simulink model "QD2_MissionCtrl_Swarm_6x_R2021a"  (R2021a)
settings: Solver=ode2  StartTime=0.0  StopTime=inf  FixedStep=0.001  RelTol=1e-3  EnableMultiTasking=on
undefined symbols (not defined in the file): datetime, Host, localhost, m, qc_get_step_size, saved_data
libraries: quarc_library x64, simulink x19, simulink_extras x1
(part 3 of 3)

== system QD2_MissionCtrl_Swarm_6x_R2021a/MISSION SERVER QDRONE SWARM/Calculate Home Pose V6/Enabled Subsystem ==
  "Pose (m, rad ) [4] " : Inport
  Enable : EnablePort
  "Home Pose (m, rad ) [4]" : Outport  VectorParamsAs1DForOutWhenUnconnected=off
  wires:
  "Pose (m, rad ) [4] "/1 -> "Home Pose (m, rad ) [4]"/1

== system QD2_MissionCtrl_Swarm_6x_R2021a/MISSION SERVER QDRONE SWARM/Calculate Home Pose V7/Enabled Subsystem ==
  "Pose (m, rad ) [4] " : Inport
  Enable : EnablePort
  "Home Pose (m, rad ) [4]" : Outport  VectorParamsAs1DForOutWhenUnconnected=off
  wires:
  "Pose (m, rad ) [4] "/1 -> "Home Pose (m, rad ) [4]"/1

== system QD2_MissionCtrl_Swarm_6x_R2021a/MISSION SERVER QDRONE SWARM/Communications Check/Triggered Subsystem ==
  note: This looks for the first falling edge to trigger a communication issue,
      | because the mission server model starts first.
  Trigger : TriggerPort  TriggerType=falling  VariantControl=Variant
  Add : Sum
  Compare To Constant : simulink/Logic and Bit Operations/Compare To Constant  relop=>=  const=1  OutDataTypeStr=boolean
  Constant : Constant
  Memory : Memory  InheritSampleTime=on
  Communication Issue (0,1) : Outport  InitialOutput=0  VectorParamsAs1DForOutWhenUnconnected=off
  wires:
  Constant/1 -> Add/1
  Memory/1 -> Add/2
  Add/1 -> Compare To Constant/1, Memory/1
  Compare To Constant/1 -> Communication Issue (0,1)/1

== system QD2_MissionCtrl_Swarm_6x_R2021a/MISSION SERVER QDRONE SWARM/Communications Check/Triggered Subsystem1 ==
  note: This looks for the first falling edge to trigger a communication issue,
      | because the mission server model starts first.
  Trigger : TriggerPort  TriggerType=falling  VariantControl=Variant
  Add : Sum
  Compare To Constant : simulink/Logic and Bit Operations/Compare To Constant  relop=>=  const=1  OutDataTypeStr=boolean
  Constant : Constant
  Memory : Memory  InheritSampleTime=on
  Communication Issue (0,1) : Outport  InitialOutput=0  VectorParamsAs1DForOutWhenUnconnected=off
  wires:
  Compare To Constant/1 -> Communication Issue (0,1)/1
  Add/1 -> Memory/1, Compare To Constant/1
  Memory/1 -> Add/2
  Constant/1 -> Add/1

== system QD2_MissionCtrl_Swarm_6x_R2021a/MISSION SERVER QDRONE SWARM/Communications Check/Triggered Subsystem2 ==
  note: This looks for the first falling edge to trigger a communication issue,
      | because the mission server model starts first.
  Trigger : TriggerPort  TriggerType=falling  VariantControl=Variant
  Add : Sum
  Compare To Constant : simulink/Logic and Bit Operations/Compare To Constant  relop=>=  const=1  OutDataTypeStr=boolean
  Constant : Constant
  Memory : Memory  InheritSampleTime=on
  Communication Issue (0,1) : Outport  InitialOutput=0  VectorParamsAs1DForOutWhenUnconnected=off
  wires:
  Constant/1 -> Add/1
  Memory/1 -> Add/2
  Add/1 -> Compare To Constant/1, Memory/1
  Compare To Constant/1 -> Communication Issue (0,1)/1

== system QD2_MissionCtrl_Swarm_6x_R2021a/MISSION SERVER QDRONE SWARM/Communications Check/Triggered Subsystem3 ==
  note: This looks for the first falling edge to trigger a communication issue,
      | because the mission server model starts first.
  Trigger : TriggerPort  TriggerType=falling  VariantControl=Variant
  Add : Sum
  Compare To Constant : simulink/Logic and Bit Operations/Compare To Constant  relop=>=  const=1  OutDataTypeStr=boolean
  Constant : Constant
  Memory : Memory  InheritSampleTime=on
  Communication Issue (0,1) : Outport  InitialOutput=0  VectorParamsAs1DForOutWhenUnconnected=off
  wires:
  Compare To Constant/1 -> Communication Issue (0,1)/1
  Add/1 -> Memory/1, Compare To Constant/1
  Memory/1 -> Add/2
  Constant/1 -> Add/1

== system QD2_MissionCtrl_Swarm_6x_R2021a/MISSION SERVER QDRONE SWARM/Communications Check/Triggered Subsystem4 ==
  note: This looks for the first falling edge to trigger a communication issue,
      | because the mission server model starts first.
  Trigger : TriggerPort  TriggerType=falling  VariantControl=Variant
  Add : Sum
  Compare To Constant : simulink/Logic and Bit Operations/Compare To Constant  relop=>=  const=1  OutDataTypeStr=boolean
  Constant : Constant
  Memory : Memory  InheritSampleTime=on
  Communication Issue (0,1) : Outport  InitialOutput=0  VectorParamsAs1DForOutWhenUnconnected=off
  wires:
  Constant/1 -> Add/1
  Memory/1 -> Add/2
  Add/1 -> Compare To Constant/1, Memory/1
  Compare To Constant/1 -> Communication Issue (0,1)/1

== system QD2_MissionCtrl_Swarm_6x_R2021a/MISSION SERVER QDRONE SWARM/Communications Check/Triggered Subsystem5 ==
  note: This looks for the first falling edge to trigger a communication issue,
      | because the mission server model starts first.
  Trigger : TriggerPort  TriggerType=falling  VariantControl=Variant
  Add : Sum
  Compare To Constant : simulink/Logic and Bit Operations/Compare To Constant  relop=>=  const=1  OutDataTypeStr=boolean
  Constant : Constant
  Memory : Memory  InheritSampleTime=on
  Communication Issue (0,1) : Outport  InitialOutput=0  VectorParamsAs1DForOutWhenUnconnected=off
  wires:
  Compare To Constant/1 -> Communication Issue (0,1)/1
  Add/1 -> Memory/1, Compare To Constant/1
  Memory/1 -> Add/2
  Constant/1 -> Add/1

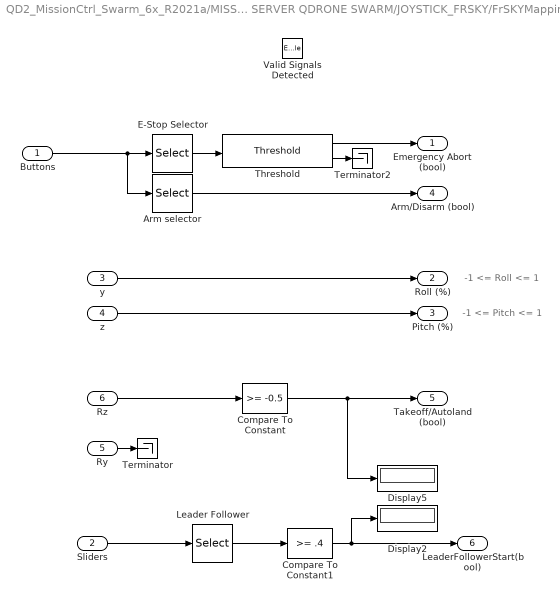
== system QD2_MissionCtrl_Swarm_6x_R2021a/MISSION SERVER QDRONE SWARM/JOYSTICK_FRSKY/FrSKYMapping ==
  note: -1 <= Roll <= 1
  note: -1 <= Pitch <= 1
  Buttons : Inport
  Sliders : Inport  Port=2
  y : Inport  Port=3
  z : Inport  Port=4
  Ry : Inport  Port=5
  Rz : Inport  Port=6
  Valid Signals Detected : EnablePort
  Arm selector : Selector  InputPortWidth=32  IndexOptions=Index vector (dialog)  Indices=[2]  OutputSizes=1
  Compare To Constant : simulink/Logic and Bit Operations/Compare To Constant  relop=>=  const=-0.5  OutDataTypeStr=boolean
  Compare To Constant1 : simulink/Logic and Bit Operations/Compare To Constant  relop=>=  const=.4  OutDataTypeStr=boolean
  Display2 : Display
  Display5 : Display
  E-Stop Selector : Selector  InputPortWidth=32  IndexOptions=Index vector (dialog)  Indices=[1]  OutputSizes=1
  Leader Follower : Selector  InputPortWidth=2  IndexOptions=Index vector (dialog)  Indices=[1]  OutputSizes=1
  Terminator : Terminator
  Terminator2 : Terminator
  Threshold : quarc_library/Discontinuities/Threshold  operator=>=  param_src=Specify via dialog  threshold=0.5  duration=0.2
      settings: SourceProductName=QUARC Targets
  Emergency Abort (bool) : Outport  VectorParamsAs1DForOutWhenUnconnected=off
  Roll (%) : Outport  Port=2  VectorParamsAs1DForOutWhenUnconnected=off
  Pitch (%) : Outport  Port=3  VectorParamsAs1DForOutWhenUnconnected=off
  "Arm/Disarm (bool) " : Outport  Port=4  VectorParamsAs1DForOutWhenUnconnected=off
  Takeoff/Autoland (bool) : Outport  Port=5  VectorParamsAs1DForOutWhenUnconnected=off
  LeaderFollowerStart(bool) : Outport  Port=6  VectorParamsAs1DForOutWhenUnconnected=off
  wires:
  Buttons/1 -> Arm selector/1, E-Stop Selector/1
  Arm selector/1 -> "Arm/Disarm (bool) "/1
  y/1 -> Roll (%)/1
  z/1 -> Pitch (%)/1
  Rz/1 -> Compare To Constant/1
  Sliders/1 -> Leader Follower/1
  E-Stop Selector/1 -> Threshold/1
  Compare To Constant/1 -> Takeoff/Autoland (bool)/1, Display5/1
  Threshold/1 -> Emergency Abort (bool)/1
  Threshold/2 -> Terminator2/1
  Leader Follower/1 -> Compare To Constant1/1
  Compare To Constant1/1 -> Display2/1, LeaderFollowerStart(bool)/1
  Ry/1 -> Terminator/1

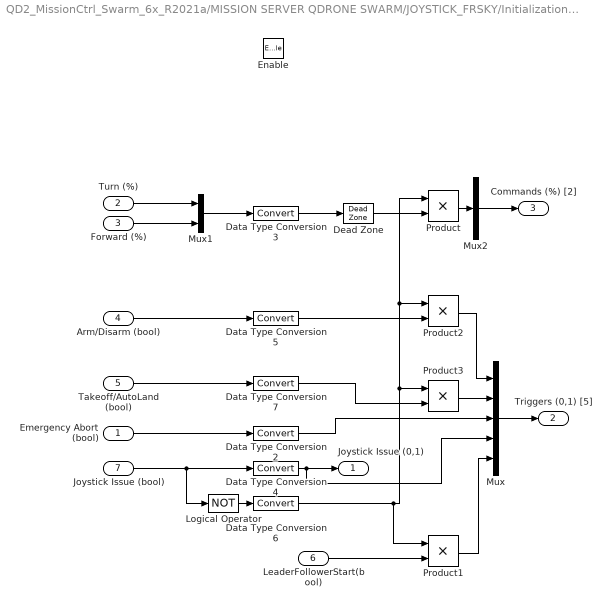
== system QD2_MissionCtrl_Swarm_6x_R2021a/MISSION SERVER QDRONE SWARM/JOYSTICK_FRSKY/Initialization and Conditioning ==
  Emergency Abort (bool) : Inport
  Turn (%) : Inport  Port=2
  Forward (%) : Inport  Port=3
  Arm/Disarm (bool) : Inport  Port=4
  Takeoff/AutoLand (bool) : Inport  Port=5
  LeaderFollowerStart(bool) : Inport  Port=6
  Joystick Issue (bool) : Inport  Port=7
  Enable : EnablePort  StatesWhenEnabling=reset
  Data Type Conversion{2..7} (6 alike) : DataTypeConversion
  Dead Zone : DeadZone  LowerValue=-0.01  UpperValue=0.01  SaturateOnIntegerOverflow=on
  Logical Operator : Logic  Operator=NOT  AllPortsSameDT=off  OutDataTypeStr=boolean
  Mux : Mux  Inputs=5
  Mux1 : Mux  Inputs=2
  Mux2 : Mux  Inputs=1
  Product{,1..3} (4 alike) : Product
  Joystick Issue (0,1) : Outport  InitialOutput=0  VectorParamsAs1DForOutWhenUnconnected=off
  Triggers (0,1) [5] : Outport  Port=2  InitialOutput=0  VectorParamsAs1DForOutWhenUnconnected=off
  Commands (%) [2] : Outport  Port=3  InitialOutput=0  VectorParamsAs1DForOutWhenUnconnected=off
  wires:
  Joystick Issue (bool)/1 -> Data Type Conversion4/1, Logical Operator/1
  Mux1/1 -> Data Type Conversion3/1
  Turn (%)/1 -> Mux1/1
  Forward (%)/1 -> Mux1/2
  Data Type Conversion4/1 -> Joystick Issue (0,1)/1, Mux/4
  Emergency Abort (bool)/1 -> Data Type Conversion2/1
  Data Type Conversion3/1 -> Dead Zone/1
  Arm/Disarm (bool)/1 -> Data Type Conversion5/1
  Mux/1 -> Triggers (0,1) [5]/1
  Data Type Conversion2/1 -> Mux/3
  Logical Operator/1 -> Data Type Conversion6/1
  Product/1 -> Mux2/1
  Dead Zone/1 -> Product/2
  Data Type Conversion6/1 -> Product3/1, Product2/1, Product/1, Product1/1
  Product2/1 -> Mux/1
  Data Type Conversion5/1 -> Product2/2
  Takeoff/AutoLand (bool)/1 -> Data Type Conversion7/1
  Product3/1 -> Mux/2
  Data Type Conversion7/1 -> Product3/2
  Mux2/1 -> Commands (%) [2]/1
  LeaderFollowerStart(bool)/1 -> Product1/2
  Product1/1 -> Mux/5

== system QD2_MissionCtrl_Swarm_6x_R2021a/MISSION SERVER QDRONE SWARM/JOYSTICK_FRSKY/Pulse Check ==
  note: For this subsystem we will count the number of new pulses. The data can be considered enabled once the count of new signals has gone beyond 2. This will enable the Initializing and conditioning subsystem.
  new : Inport
  Compare : quarc_library/Logic Operations/Compare  operator=>=  output_data_type=boolean
      settings: SourceProductName=QUARC Targets
  Pulse Check : Constant
  "pulse count " : Subsystem  TreatAsAtomicUnit=on
  signal enable : Outport  InitialOutput=0  VectorParamsAs1DForOutWhenUnconnected=off
  wires:
  Compare/1 -> signal enable/1
  Pulse Check/1 -> Compare/2
  new/1 -> "pulse count "/Trigger
  "pulse count "/1(Number of Pulses) -> Compare/1

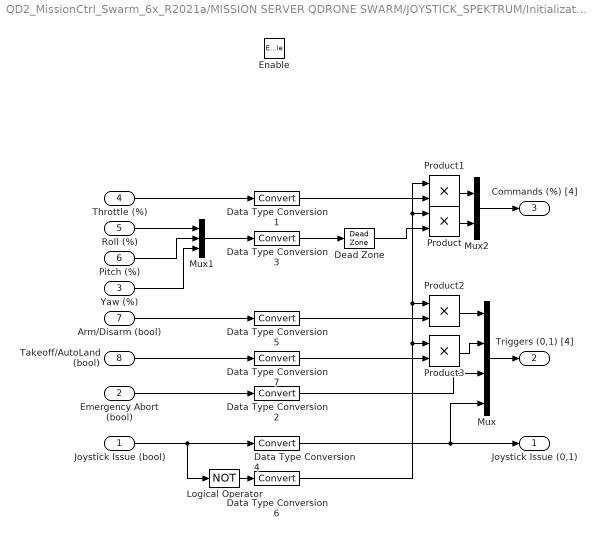
== system QD2_MissionCtrl_Swarm_6x_R2021a/MISSION SERVER QDRONE SWARM/JOYSTICK_SPEKTRUM/Initialization and Conditioning ==
  Joystick Issue (bool) : Inport
  Emergency Abort (bool) : Inport  Port=2
  Yaw (%) : Inport  Port=3
  Throttle (%) : Inport  Port=4
  Roll (%) : Inport  Port=5
  Pitch (%) : Inport  Port=6
  Arm/Disarm (bool) : Inport  Port=7
  Takeoff/AutoLand (bool) : Inport  Port=8
  Enable : EnablePort  StatesWhenEnabling=reset
  Data Type Conversion{1..7} (7 alike) : DataTypeConversion
  Dead Zone : DeadZone  LowerValue=-0.01  UpperValue=0.01  SaturateOnIntegerOverflow=on
  Logical Operator : Logic  Operator=NOT  AllPortsSameDT=off  OutDataTypeStr=boolean
  Mux : Mux
  Mux1 : Mux  Inputs=3
  Mux2 : Mux  Inputs=2
  Product{,1..3} (4 alike) : Product
  Joystick Issue (0,1) : Outport  InitialOutput=0  VectorParamsAs1DForOutWhenUnconnected=off
  Triggers (0,1) [4] : Outport  Port=2  InitialOutput=0  VectorParamsAs1DForOutWhenUnconnected=off
  Commands (%) [4] : Outport  Port=3  InitialOutput=0  VectorParamsAs1DForOutWhenUnconnected=off
  wires:
  Mux2/1 -> Commands (%) [4]/1
  Data Type Conversion7/1 -> Product3/2
  Product3/1 -> Mux/2
  Takeoff/AutoLand (bool)/1 -> Data Type Conversion7/1
  Data Type Conversion5/1 -> Product2/2
  Product2/1 -> Mux/1
  Data Type Conversion6/1 -> Product3/1, Product2/1, Product/1, Product1/1
  Dead Zone/1 -> Product/2
  Data Type Conversion1/1 -> Product1/2
  Product1/1 -> Mux2/1
  Product/1 -> Mux2/2
  Logical Operator/1 -> Data Type Conversion6/1
  Data Type Conversion2/1 -> Mux/3
  Mux/1 -> Triggers (0,1) [4]/1
  Arm/Disarm (bool)/1 -> Data Type Conversion5/1
  Data Type Conversion3/1 -> Dead Zone/1
  Emergency Abort (bool)/1 -> Data Type Conversion2/1
  Data Type Conversion4/1 -> Joystick Issue (0,1)/1, Mux/4
  Yaw (%)/1 -> Mux1/3
  Pitch (%)/1 -> Mux1/2
  Roll (%)/1 -> Mux1/1
  Throttle (%)/1 -> Data Type Conversion1/1
  Mux1/1 -> Data Type Conversion3/1
  Joystick Issue (bool)/1 -> Logical Operator/1, Data Type Conversion4/1

== system QD2_MissionCtrl_Swarm_6x_R2021a/MISSION SERVER QDRONE SWARM/JOYSTICK_SPEKTRUM/Pulse Check ==
  note: For this subsystem we will count the number of new pulses. The data can be considered enabled once the count of new signals has gone beyond 2. This will enable the Initializing and conditioning subsystem.
  new : Inport
  Compare : quarc_library/Logic Operations/Compare  operator=>  output_data_type=boolean
      settings: SourceProductName=QUARC Targets
  Pulse Check : Constant  Value=2
  "pulse count " : Subsystem  TreatAsAtomicUnit=on
  signal enable : Outport  InitialOutput=0  VectorParamsAs1DForOutWhenUnconnected=off
  wires:
  Compare/1 -> signal enable/1
  Pulse Check/1 -> Compare/2
  new/1 -> "pulse count "/Trigger
  "pulse count "/1(Number of Pulses) -> Compare/1

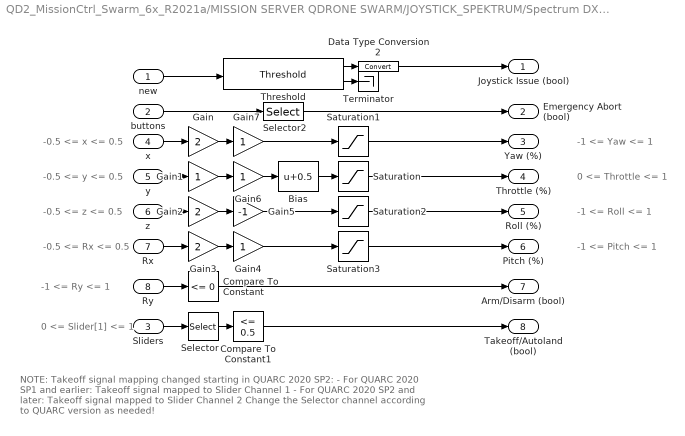
== system QD2_MissionCtrl_Swarm_6x_R2021a/MISSION SERVER QDRONE SWARM/JOYSTICK_SPEKTRUM/Spectrum DXe Mapping ==
  note: NOTE: Takeoff signal mapping changed starting in QUARC 2020 SP2:
      |
      | - For QUARC 2020 SP1 and earlier: Takeoff signal mapped to Slider Channel 1
      | - For QUARC 2020 SP2 and later: Takeoff signal mapped to Slider Channel 2
      |
      | Change the Selector channel according to QUARC version as needed!
  note: -1 <= Ry <= 1
  note: 0 <= Slider[1] <= 1
  note: -1 <= Pitch <= 1
  note: -0.5 <= Rx <= 0.5
  note: -1 <= Roll <= 1
  note: -0.5 <= z <= 0.5
  note: 0 <= Throttle <= 1
  note: -0.5 <= y <= 0.5
  note: -1 <= Yaw <= 1
  note: -0.5 <= x <= 0.5
  new : Inport
  buttons : Inport  Port=2
  Sliders : Inport  Port=3
  x : Inport  Port=4
  y : Inport  Port=5
  z : Inport  Port=6
  Rx : Inport  Port=7
  Ry : Inport  Port=8
  Bias : Bias  Bias=0.5
  Compare To Constant : simulink/Logic and Bit Operations/Compare To Constant  relop=<=  const=0  OutDataTypeStr=boolean
  Compare To Constant1 : simulink/Logic and Bit Operations/Compare To Constant  relop=<=  const=0.5  OutDataTypeStr=boolean
  Data Type Conversion2 : DataTypeConversion
  Gain : Gain  Gain=2
  Gain{1,4,6..7} (4 alike) : Gain
  Gain2 : Gain  Gain=2
  Gain3 : Gain  Gain=2
  Gain5 : Gain  Gain=-1
  Saturation : Saturate  UpperLimit=1  LowerLimit=0
  Saturation1 : Saturate  UpperLimit=1  LowerLimit=-1
  Saturation2 : Saturate  UpperLimit=1  LowerLimit=-1
  Saturation3 : Saturate  UpperLimit=1  LowerLimit=-1
  Selector : Selector  InputPortWidth=2  IndexOptions=Index vector (dialog)  Indices=[2]  OutputSizes=1
  Selector2 : Selector  InputPortWidth=32  IndexOptions=Index vector (dialog)  Indices=[1]  OutputSizes=1
  Terminator : Terminator
  Threshold : quarc_library/Discontinuities/Threshold  operator===  param_src=Specify via dialog  threshold=0  duration=1
      settings: SourceProductName=QUARC Targets
  Joystick Issue (bool) : Outport  VectorParamsAs1DForOutWhenUnconnected=off
  Emergency Abort (bool) : Outport  Port=2  VectorParamsAs1DForOutWhenUnconnected=off
  Yaw (%) : Outport  Port=3  VectorParamsAs1DForOutWhenUnconnected=off
  Throttle (%) : Outport  Port=4  VectorParamsAs1DForOutWhenUnconnected=off
  Roll (%) : Outport  Port=5  VectorParamsAs1DForOutWhenUnconnected=off
  Pitch (%) : Outport  Port=6  VectorParamsAs1DForOutWhenUnconnected=off
  "Arm/Disarm (bool) " : Outport  Port=7  VectorParamsAs1DForOutWhenUnconnected=off
  Takeoff/Autoland (bool) : Outport  Port=8  VectorParamsAs1DForOutWhenUnconnected=off
  wires:
  Data Type Conversion2/1 -> Joystick Issue (bool)/1
  new/1 -> Threshold/1
  Threshold/1 -> Data Type Conversion2/1
  Selector2/1 -> Emergency Abort (bool)/1
  Threshold/2 -> Terminator/1
  buttons/1 -> Selector2/1
  Compare To Constant1/1 -> Takeoff/Autoland (bool)/1
  Rx/1 -> Gain3/1
  y/1 -> Gain1/1
  Ry/1 -> Compare To Constant/1
  x/1 -> Gain/1
  z/1 -> Gain2/1
  Gain4/1 -> Saturation3/1
  Gain1/1 -> Gain6/1
  Gain2/1 -> Gain5/1
  Bias/1 -> Saturation/1
  Saturation2/1 -> Roll (%)/1
  Gain3/1 -> Gain4/1
  Gain/1 -> Gain7/1
  Saturation1/1 -> Yaw (%)/1
  Gain6/1 -> Bias/1
  Sliders/1 -> Selector/1
  Saturation/1 -> Throttle (%)/1
  Gain5/1 -> Saturation2/1
  Selector/1 -> Compare To Constant1/1
  Gain7/1 -> Saturation1/1
  Saturation3/1 -> Pitch (%)/1
  Compare To Constant/1 -> "Arm/Disarm (bool) "/1

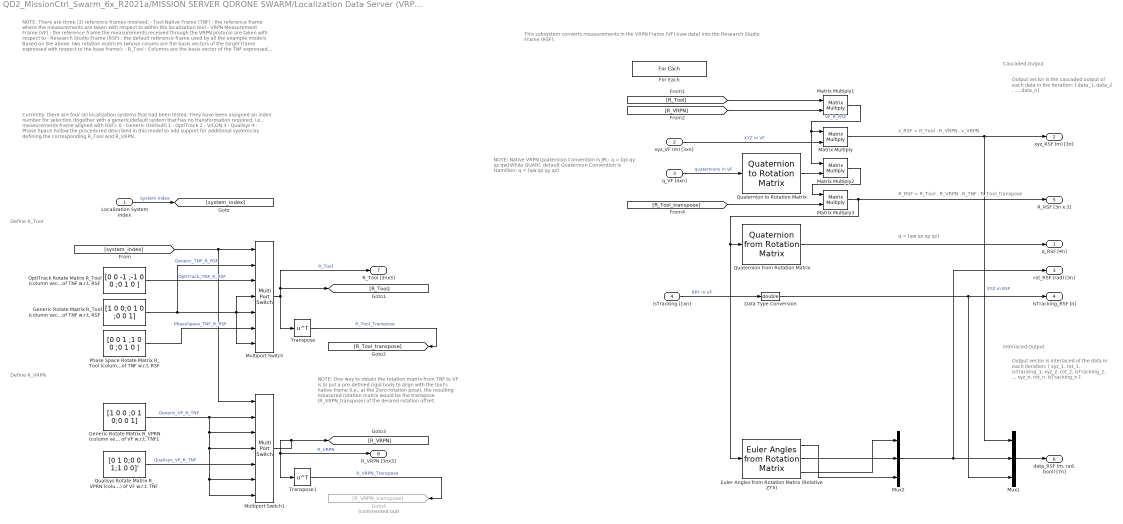
== system QD2_MissionCtrl_Swarm_6x_R2021a/MISSION SERVER QDRONE SWARM/Localization Data Server (VRPN) /For Each Subsystem (Convention Correction: Motive Frame to Research Studio Frame)1 ==
  note: R_RSF = R_Tool . R_VRPN . R_TNF . R_Tool_transpose
  note: v_RSF = R_Tool . R_VRPN . v_VRPN
  note: Define R_VRPN
  note: Currently, there are four (4) localization systems that had been tested. They have been assigned an index number for selection (together with a generic/default system that has no transformation required, i.e., measurements frame aligned with RSF):
      |
      | 0 - Generic (Default)
      | 1 - OptiTrack
      | 2 - VICON
      | 3 - Qualisys
      | 4 - Phase Space
      |
      | Follow the procedured described in this model to add support for additional systems by defining the corresponding R_Tool and R_VRPN .
  note: Define R_Tool
  note: NOTE:
      | There are three (3) reference frames involved:
      |
      | - Tool Native Frame (TNF) : the reference frame where the measurements are taken with respect to within the localization tool
      | - VRPN Measurement Frame (VF) : the reference frame the measurements received through the VRPN protocol are taken with respect to
      | - Research Studio Frame (RSF) : the default reference frame used by all the example models
      |
      | Based on the above, two rotation matrices (whose colums are the basis vectors of the target frame expressed with respect to the base frame):
      |
      | - R_Tool : Columns are the basis vector of the TNF expressed with respect to the RSF
      | - R_VPRN : Columns are the basis vector of the VRPN frame with respect to the TNF
      |
      | If all of the reference are aligned, then both R_Tool and R_VRPN will be a 3x3 identity matrices.
  note: NOTE:
      | One way to obtain the rotation matrix from TNF to VF
      | is to put a pre-defined rigid body to align with the tool's
      | native frame (i.e., at the Zero rotation pose), the resulting
      | measured rotation matrix would be the transpose (R_VRPN_transpose) of the desired rotation
      | offset.
  note: NOTE: Native VRPN Quaternion Convention is JPL:
      | q = [qx qy qz qw]
      |
      | While QUARC default Quaternion Convention is Hamilton:
      | q = [qw qx qy qz]
  note: Output vector is interlaced of the data
      | in each iteration:
      |
      | [ xyz_1, rot_1, isTracking_1,
      |   xyz_2, rot_2, isTracking_2,
      |   ...
      |   xyz_n, rot_n, isTracking_n ]
  note: Interlaced Output
  note: Output vector is the cascaded output of
      | each data in the iteration:
      | [ data_1, data_2 , ..., data_n]
  note: Cascaded Output
  note: q = [qw qx qy qz]
  note: This subsystem converts measurements in the VRPN Frame (VF) (raw data) into the Research Studio Frame (RSF).
  Localization System Index : Inport
  xyz_VF (m) [3xn] : Inport  Port=2  Partition=on  PartitionDimension=2  PartitionWidth=1  PartitionOffset=0
  q_VF [4xn] : Inport  Port=3  Partition=on  PartitionDimension=2  PartitionWidth=1  PartitionOffset=0
  isTracking [1xn] : Inport  Port=4  Partition=on  PartitionDimension=2  PartitionWidth=1  PartitionOffset=0
  " Generic Rotate Matrix R_VPRN (column vectors are basis vectors) of VF w.r.t. TNF1" : Constant  Value=[1 0 0 ;0 1 0;0 0 1]  VectorParams1D=off
  " Qualisys Rotate Matrix R_VPRN (column vectors are basis vectors) of VF w.r.t. TNF" : Constant  Value=[0 1 0;0 0 1;1 0 0]'  VectorParams1D=off
  Data Type Conversion : DataTypeConversion  OutDataTypeStr=double
  Euler Angles from Rotation Matrix (Relative ZYX) : quarc_library/Math Operations/Matrices/Euler Angles from Rotation Matrix  menu_order=Relative Z-Y-X
      settings: SourceProductName=QUARC Targets
  For Each : ForEach  DisableCoverage=on
  Generic Rotate Matrix R_Tool (column vectors are basis vectors) of TNF w.r.t. RSF : Constant  Value=[1 0 0;0 1 0 ;0 0 1]  VectorParams1D=off
  Goto4 : Goto  Commented=on  GotoTag=R_VRPN_transpose
  Matrix Multiply{,1..3} (4 alike) : Product  Multiplication=Matrix(*)
  Multiport Switch : MultiPortSwitch  DataPortOrder=Zero-based contiguous  Inputs=5  DataPortForDefault=Additional data port  DiagnosticForDefault=None  zeroidx=on
  Multiport Switch1 : MultiPortSwitch  DataPortOrder=Zero-based contiguous  Inputs=5  DataPortForDefault=Additional data port  DiagnosticForDefault=None  zeroidx=on
  Mux1 : Mux  Inputs=3
  Mux2 : Mux  Inputs=3
  OptiTrack Rotate Matrix R_Tool (column vectors are basis vectors) of TNF w.r.t. RSF : Constant  Value=[0 0 -1 ;-1 0 0 ;0 1 0 ]  VectorParams1D=off
  Phase Space Rotate Matrix R_Tool (column vectors are basis vectors) of TNF w.r.t. RSF : Constant  Value=[0 0 1 ;1 0 0 ;0 1 0 ]  VectorParams1D=off
  Quaternion from Rotation Matrix : quarc_library/Math Operations/Quaternions/Quaternion from Rotation Matrix
      settings: SourceProductName=QUARC Targets
  Quaternion to Rotation Matrix : quarc_library/Math Operations/Quaternions/Quaternion to Rotation Matrix
      settings: SourceProductName=QUARC Targets
  Transpose : Math  Operator=transpose  SaturateOnIntegerOverflow=on
  Transpose1 : Math  Operator=transpose  SaturateOnIntegerOverflow=on
  q_RSF [4n] : Outport  ConcatenationDimension=1
  xyz_RSF (m) [3n] : Outport  Port=2  ConcatenationDimension=1
  rot_RSF (rad) [3n] : Outport  Port=3  ConcatenationDimension=1
  isTracking_RSF [n] : Outport  Port=4  ConcatenationDimension=1
  R_RSF [3n x 3] : Outport  Port=5  ConcatenationDimension=1
  "data_RSF (m, rad, bool) [7n]" : Outport  Port=6  ConcatenationDimension=1
  R_Tool [3nx3] : Outport  Port=7  ConcatenationDimension=1
  R_VRPN [3nx3] : Outport  Port=8  ConcatenationDimension=1
  wires:
  q_VF [4xn]/1 -> Quaternion to Rotation Matrix/1  "quaternions in VF"
  Matrix Multiply/1 -> xyz_RSF (m) [3n]/1, Mux1/1  "XYZ in RSF"
  xyz_VF (m) [3xn]/1 -> Matrix Multiply/2  "XYZ in VF"
  isTracking [1xn]/1 -> Data Type Conversion/1  "RPY in VF"
  Mux1/1 -> "data_RSF (m, rad, bool) [7n]"/1
  Data Type Conversion/1 -> Mux1/3, isTracking_RSF [n]/1
  Euler Angles from Rotation Matrix (Relative ZYX)/3 -> Mux2/1
  Euler Angles from Rotation Matrix (Relative ZYX)/1 -> Mux2/3
  Euler Angles from Rotation Matrix (Relative ZYX)/2 -> Mux2/2
  Mux2/1 -> Mux1/2, rot_RSF (rad) [3n]/1
  Quaternion to Rotation Matrix/1 -> Matrix Multiply2/2
  Matrix Multiply2/1 -> Matrix Multiply3/1
  Quaternion from Rotation Matrix/1 -> q_RSF [4n]/1
  Generic Rotate Matrix R_Tool (column vectors are basis vectors) of TNF w.r.t. RSF/1 -> Multiport Switch/4, Multiport Switch/5, Multiport Switch/7, Multiport Switch/2  "Generic_TNF_R_RSF"
  OptiTrack Rotate Matrix R_Tool (column vectors are basis vectors) of TNF w.r.t. RSF/1 -> Multiport Switch/3  "OptiTrack_TNF_R_RSF"
  " Generic Rotate Matrix R_VPRN (column vectors are basis vectors) of VF w.r.t. TNF1"/1 -> Multiport Switch1/6, Multiport Switch1/7, Multiport Switch1/4, Multiport Switch1/3, Multiport Switch1/2  "Generic_VF_R_TNF"
  " Qualisys Rotate Matrix R_VPRN (column vectors are basis vectors) of VF w.r.t. TNF"/1 -> Multiport Switch1/5  "Qualisys_VF_R_TNF"
  [system_index] -> Multiport Switch1/1, Multiport Switch/1
  Multiport Switch/1 -> R_Tool [3nx3]/1, [R_Tool], Transpose/1  "R_Tool"
  Transpose/1 -> [R_Tool_transpose]  "R_Tool_Transpose"
  Multiport Switch1/1 -> R_VRPN [3nx3]/1, Transpose1/1, [R_VRPN]  "R_VRPN"
  Transpose1/1 -> Goto4/1  "R_VRPN_Transpose"
  [R_Tool] -> Matrix Multiply1/1
  [R_VRPN] -> Matrix Multiply1/2
  Matrix Multiply1/1 -> Matrix Multiply2/1, Matrix Multiply/1  "VF_R_RSF"
  [R_Tool_transpose] -> Matrix Multiply3/2
  Matrix Multiply3/1 -> Euler Angles from Rotation Matrix (Relative ZYX)/1, Quaternion from Rotation Matrix/1, R_RSF [3n x 3]/1
  Localization System Index/1 -> [system_index]  "System Index"
  Phase Space Rotate Matrix R_Tool (column vectors are basis vectors) of TNF w.r.t. RSF/1 -> Multiport Switch/6  "PhaseSpace_TNF_R_RSF"

== system QD2_MissionCtrl_Swarm_6x_R2021a/MISSION SERVER QDRONE SWARM/JOYSTICK_FRSKY/Pulse Check/pulse count  ==
  Trigger : TriggerPort  VariantControl=Variant
  Constant1 : Constant  Value=0
  Increment Stored Integer : simulink/Additional Math & Discrete/Additional Math: Increment - Decrement/Increment Stored Integer
  Sum : Sum  Inputs=|++
  Unit Delay : UnitDelay  SampleTime=-1  HasFrameUpgradeWarning=on
  Number of Pulses : Outport  VectorParamsAs1DForOutWhenUnconnected=off
  wires:
  Constant1/1 -> Sum/1
  Sum/1 -> Increment Stored Integer/1
  Unit Delay/1 -> Sum/2
  Increment Stored Integer/1 -> Unit Delay/1, Number of Pulses/1

== system QD2_MissionCtrl_Swarm_6x_R2021a/MISSION SERVER QDRONE SWARM/JOYSTICK_SPEKTRUM/Pulse Check/pulse count  ==
  Trigger : TriggerPort  VariantControl=Variant
  Constant1 : Constant  Value=0
  Increment Stored Integer : simulink/Additional Math & Discrete/Additional Math: Increment - Decrement/Increment Stored Integer
  Sum : Sum  Inputs=|++
  Unit Delay : UnitDelay  SampleTime=-1  HasFrameUpgradeWarning=on
  Number of Pulses : Outport  VectorParamsAs1DForOutWhenUnconnected=off
  wires:
  Constant1/1 -> Sum/1
  Sum/1 -> Increment Stored Integer/1
  Unit Delay/1 -> Sum/2
  Increment Stored Integer/1 -> Unit Delay/1, Number of Pulses/1

== matlab function QD2_MissionCtrl_Swarm_6x_R2021a/MISSION SERVER QDRONE SWARM/Extract Vehicle Data 1/Extract Object Data ==
  data: data input; position output; orientation output; index input; tracking output

function [position, orientation, tracking] = fcn(data, index)

n = length(data)/7;


% position = data((index-1)*3 + 1: (index-1)*3 + 3);
% orientation = data( 3*n + 3*(index-1) + 1: 3*n + 3*(index-1) + 3);
% tracking = data(end-n+index - 1);


if (index<=0)||(index>n)
    position = zeros(1,3); orientation = zeros(1,3); tracking = 0;
else
    position = [data(index*7 -6) data(index*7 -5) data(index*7 -4)];
    orientation = [data(index*7 -3) data(index*7 -2) data(index*7 -1)];
    tracking = data(index*7);
end

== matlab function QD2_MissionCtrl_Swarm_6x_R2021a/MISSION SERVER QDRONE SWARM/Extract Vehicle Data 2/Extract Object Data ==
  data: data input; position output; orientation output; index input; tracking output

function [position, orientation, tracking] = fcn(data, index)

n = length(data)/7;


% position = data((index-1)*3 + 1: (index-1)*3 + 3);
% orientation = data( 3*n + 3*(index-1) + 1: 3*n + 3*(index-1) + 3);
% tracking = data(end-n+index - 1);


if (index<=0)||(index>n)
    position = zeros(1,3); orientation = zeros(1,3); tracking = 0;
else
    position = [data(index*7 -6) data(index*7 -5) data(index*7 -4)];
    orientation = [data(index*7 -3) data(index*7 -2) data(index*7 -1)];
    tracking = data(index*7);
end

== matlab function QD2_MissionCtrl_Swarm_6x_R2021a/MISSION SERVER QDRONE SWARM/Extract Vehicle Data 3/Extract Object Data ==
  data: data input; position output; orientation output; index input; tracking output

function [position, orientation, tracking] = fcn(data, index)

n = length(data)/7;


% position = data((index-1)*3 + 1: (index-1)*3 + 3);
% orientation = data( 3*n + 3*(index-1) + 1: 3*n + 3*(index-1) + 3);
% tracking = data(end-n+index - 1);


if (index<=0)||(index>n)
    position = zeros(1,3); orientation = zeros(1,3); tracking = 0;
else
    position = [data(index*7 -6) data(index*7 -5) data(index*7 -4)];
    orientation = [data(index*7 -3) data(index*7 -2) data(index*7 -1)];
    tracking = data(index*7);
end

== matlab function QD2_MissionCtrl_Swarm_6x_R2021a/MISSION SERVER QDRONE SWARM/n vehicles Circular Trajectories/generate vector of 0s for Yaw ==
  data: u input; y output
function y = fcn(u)

y = 0.*u;

== matlab function QD2_MissionCtrl_Swarm_6x_R2021a/MISSION SERVER QDRONE SWARM/Extract Vehicle Data 4/Extract Object Data ==
  data: data input; position output; orientation output; index input; tracking output

function [position, orientation, tracking] = fcn(data, index)

n = length(data)/7;


% position = data((index-1)*3 + 1: (index-1)*3 + 3);
% orientation = data( 3*n + 3*(index-1) + 1: 3*n + 3*(index-1) + 3);
% tracking = data(end-n+index - 1);


if (index<=0)||(index>n)
    position = zeros(1,3); orientation = zeros(1,3); tracking = 0;
else
    position = [data(index*7 -6) data(index*7 -5) data(index*7 -4)];
    orientation = [data(index*7 -3) data(index*7 -2) data(index*7 -1)];
    tracking = data(index*7);
end

== matlab function QD2_MissionCtrl_Swarm_6x_R2021a/MISSION SERVER QDRONE SWARM/Extract Vehicle Data 5/Extract Object Data ==
  data: data input; position output; orientation output; index input; tracking output

function [position, orientation, tracking] = fcn(data, index)

n = length(data)/7;


% position = data((index-1)*3 + 1: (index-1)*3 + 3);
% orientation = data( 3*n + 3*(index-1) + 1: 3*n + 3*(index-1) + 3);
% tracking = data(end-n+index - 1);


if (index<=0)||(index>n)
    position = zeros(1,3); orientation = zeros(1,3); tracking = 0;
else
    position = [data(index*7 -6) data(index*7 -5) data(index*7 -4)];
    orientation = [data(index*7 -3) data(index*7 -2) data(index*7 -1)];
    tracking = data(index*7);
end

== matlab function QD2_MissionCtrl_Swarm_6x_R2021a/MISSION SERVER QDRONE SWARM/Extract Vehicle Data 6/Extract Object Data ==
  data: data input; position output; orientation output; index input; tracking output

function [position, orientation, tracking] = fcn(data, index)

n = length(data)/7;


% position = data((index-1)*3 + 1: (index-1)*3 + 3);
% orientation = data( 3*n + 3*(index-1) + 1: 3*n + 3*(index-1) + 3);
% tracking = data(end-n+index - 1);


if (index<=0)||(index>n)
    position = zeros(1,3); orientation = zeros(1,3); tracking = 0;
else
    position = [data(index*7 -6) data(index*7 -5) data(index*7 -4)];
    orientation = [data(index*7 -3) data(index*7 -2) data(index*7 -1)];
    tracking = data(index*7);
end

== matlab function QD2_MissionCtrl_Swarm_6x_R2021a/Communication V6/Detect Communication loss/MATLAB Function ==
  data: time input; stream_connection_loss output; state input; error input
function stream_connection_loss  = fcn(time, state, error)

stream_connection_loss = 0;
if time > 1
    if ~((state == 2)&&(error >= 0))
        % stream connection is not established correctly
        stream_connection_loss = 1;
    end
end

== matlab function QD2_MissionCtrl_Swarm_6x_R2021a/MISSION SERVER QDRONE SWARM/n vehicles Circular Trajectories/generate vector of 1s ==
  data: u input; y output
function y = fcn(u)

y = 0.*u + 1;

== matlab function QD2_MissionCtrl_Swarm_6x_R2021a/MISSION SERVER QDRONE SWARM/n vehicles Circular Trajectories/variable size reshape ==
  data: u input; y output
function y = fcn(u)
y = u;
num = length(u)/4;
for i = 1:4
    for j = 1:num
        y(4*(j-1) + i) = u(j + num*(i-1));
    end
end

== matlab function QD2_MissionCtrl_Swarm_6x_R2021a/Communication V1/Detect Communication loss/MATLAB Function ==
  data: time input; stream_connection_loss output; state input; error input
function stream_connection_loss  = fcn(time, state, error)

stream_connection_loss = 0;
if time > 1
    if ~((state == 2)&&(error >= 0))
        % stream connection is not established correctly
        stream_connection_loss = 1;
    end
end

== matlab function QD2_MissionCtrl_Swarm_6x_R2021a/Communication V2/Detect Communication loss/MATLAB Function ==
  data: time input; stream_connection_loss output; state input; error input
function stream_connection_loss  = fcn(time, state, error)

stream_connection_loss = 0;
if time > 1
    if ~((state == 2)&&(error >= 0))
        % stream connection is not established correctly
        stream_connection_loss = 1;
    end
end

== matlab function QD2_MissionCtrl_Swarm_6x_R2021a/Communication V3/Detect Communication loss/MATLAB Function ==
  data: time input; stream_connection_loss output; state input; error input
function stream_connection_loss  = fcn(time, state, error)

stream_connection_loss = 0;
if time > 1
    if ~((state == 2)&&(error >= 0))
        % stream connection is not established correctly
        stream_connection_loss = 1;
    end
end

== matlab function QD2_MissionCtrl_Swarm_6x_R2021a/Communication V4/Detect Communication loss/MATLAB Function ==
  data: time input; stream_connection_loss output; state input; error input
function stream_connection_loss  = fcn(time, state, error)

stream_connection_loss = 0;
if time > 1
    if ~((state == 2)&&(error >= 0))
        % stream connection is not established correctly
        stream_connection_loss = 1;
    end
end

== matlab function QD2_MissionCtrl_Swarm_6x_R2021a/Communication V5/Detect Communication loss/MATLAB Function ==
  data: time input; stream_connection_loss output; state input; error input
function stream_connection_loss  = fcn(time, state, error)

stream_connection_loss = 0;
if time > 1
    if ~((state == 2)&&(error >= 0))
        % stream connection is not established correctly
        stream_connection_loss = 1;
    end
end

== matlab function QD2_MissionCtrl_Swarm_6x_R2021a/MISSION SERVER QDRONE SWARM/Extract Vehicle Data 7/Extract Object Data ==
  data: data input; position output; orientation output; index input; tracking output
function [position, orientation, tracking] = fcn(data, index)

n = length(data)/7;

if (index<=0)||(index>n)
    position = zeros(1,3); orientation = zeros(1,3); tracking = 0;
else
    position = [data(index*3-2), data(index*3-1), data(index*3)];
    orientation = [data((index+n)*3 - 2), data((index+n)*3 - 1), data((index+n)*3)];
    tracking = data(index + (n*6));
end
